simulink model "on_off_2022a"  (R2022a)
settings: Solver=ode4  StartTime=0.0  StopTime=1500  FixedStep=0.1  RelTol=1e-3  EnableMultiTasking=on
libraries: arduinolib x4
settings Model: ExtModeTrigDuration=2  Creator=user  LastModifiedBy=manur
settings SolverCC: AlgebraicLoopSolver=TrustRegion
settings DataIOCC: ReturnWorkspaceOutputs=off
settings OptimizationCC: EnhancedBackFolding=on  PassReuseOutputArgsAs=Individual arguments  MaxStackSize=64  OptimizeBlockOrder=speed  DifferentSizesBufferReuse=on  OptimizationCustomize=off  EfficientTunableParamExpr=on
settings DebuggingCC: ParameterTunabilityLossMsg=error  UnconnectedInputMsg=warning  UnconnectedOutputMsg=warning  UnconnectedLineMsg=warning  SFMachineParentedDataDiag=warning  ArithmeticOperatorsInVariantConditions=warning
settings HardwareCC: ProdBitPerInt=16  ProdBitPerPointer=16  ProdBitPerSizeT=16  ProdBitPerPtrDiffT=16  ProdLargestAtomicFloat=None  ProdWordSize=8  ProdHWDeviceType=Atmel->AVR
settings SFSimCC: SimUseLocalCustomCode=off  MATLABDynamicMemAlloc=off  CustomCodeUndefinedFunction=UseInterfaceOnly
settings SFSimCC: SimCustomInitializer=|
  | analogWrite(9, 0);
  | analogWrite(10, 0);
  | delay(1);
settings SFSimCC: SimCustomTerminator=|
  | analogWrite(9, 0);
  | analogWrite(10, 0);
  | delay(1);
settings RTWCC: SystemTargetFile=ert.tlc  HardwareBoard=Arduino Uno  TemplateMakefile=ert_default_tmf  GenerateReport=on  RTWUseLocalCustomCode=off  RTWUseSimCustomCode=on  Toolchain=Arduino AVR  BuildConfiguration=Faster Runs  IncludeHyperlinkInReport=on  LaunchReport=on  GenerateTraceInfo=on  GenerateTraceReport=on  GenerateTraceReportSl=on  GenerateTraceReportSf=on  GenerateTraceReportEml=on  DLArmComputeVersion=19.05
settings RTWCC: CustomInitializer=|
  | analogWrite(9, 0);
  | analogWrite(10, 0);
  | delay(1);
settings RTWCC: CustomTerminator=|
  | analogWrite(9, 0);
  | analogWrite(10, 0);
  | delay(1);
settings CodeAppCC: ForceParamTrailComments=on  IgnoreCustomStorageClasses=off  OperatorAnnotations=on  SimulinkDataObjDesc=on  SFDataObjDesc=on  InsertBlockDesc=on
settings ERTTargetCC: SupportContinuousTime=on  SupportVariableSizeSignals=on  ExtMode=on  ExtModeMexArgs='127.0.0.1' 0 17725

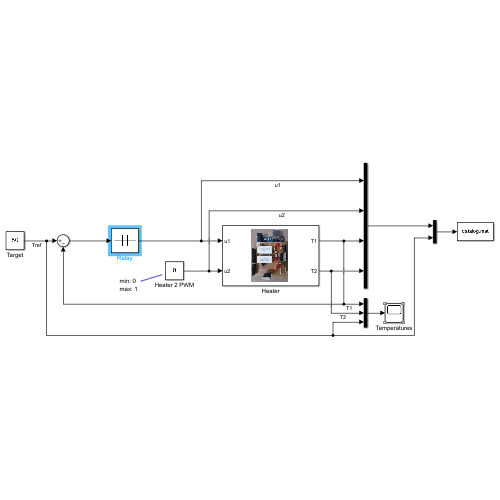
[thumbnail: Simulink's stored preview of the top-level diagram]
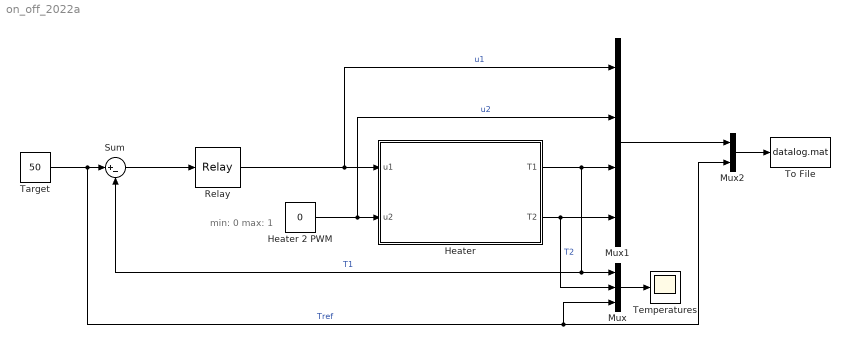
== system on_off_2022a ==
  note: min: 0
      | max: 1
  Heater : Subsystem
      mask Display: image('$imagefile'); % Use "Edit Image" on toolstrip to change.
  Heater 2 PWM : Constant  Value=0
  Mux : Mux  Inputs=3
  Mux1 : Mux
  Mux2 : Mux  Inputs=2
  Relay : Relay  OnSwitchValue=2  OffSwitchValue=-2  OnOutputValue=0.7
  Sum : Sum  Inputs=|+-
  Target : Constant  Value=50
  Temperatures : Scope
  To File : ToFile  Filename=datalog.mat  MatrixName=datalog
  wires:
  Mux1/1 -> Mux2/1
  Heater/2(T2) -> Mux/2, Mux1/4  "T2"
  Heater/1(T1) -> Mux/1, Sum/2, Mux1/3  "T1"
  Relay/1 -> Mux1/1, Heater/1(u1)  "u1"
  Mux/1 -> Temperatures/1
  Heater 2 PWM/1 -> Mux1/2, Heater/2(u2)  "u2"
  Sum/1 -> Relay/1
  Target/1 -> Mux2/2, Mux/3, Sum/1  "Tref"
  Mux2/1 -> To File/1

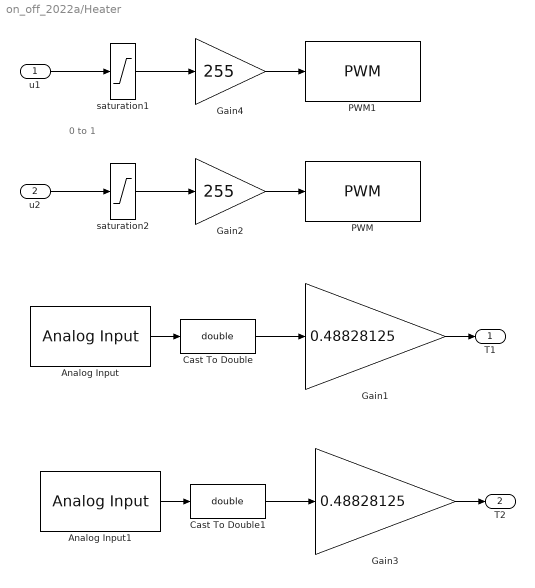
== system on_off_2022a/Heater ==
  note: 0 to 1
  u1 : Inport
  u2 : Inport  Port=2
  Analog Input : arduinolib/Analog Input  pinNumber=0  ReadResultsOnly=off  ConversionTriggerSource=Software  ExternalTriggerType=uint32(0)  OutputDataType=uint16  EnableConversionCompleteNotify=off  EnableOuputStatus=off  SampleTime=-1  blockPlatform=arduino
  Analog Input1 : arduinolib/Analog Input  pinNumber=1  ReadResultsOnly=off  ConversionTriggerSource=Software  ExternalTriggerType=uint32(0)  OutputDataType=uint16  EnableConversionCompleteNotify=off  EnableOuputStatus=off  SampleTime=-1  blockPlatform=arduino
  Cast To Double : DataTypeConversion  OutDataTypeStr=double  SaturateOnIntegerOverflow=off  RndMeth=Floor
  Cast To Double1 : DataTypeConversion  OutDataTypeStr=double  SaturateOnIntegerOverflow=off  RndMeth=Floor
  Gain1 : Gain  Gain=0.48828125
  Gain2 : Gain  Gain=255
  Gain3 : Gain  Gain=0.48828125
  Gain4 : Gain  Gain=255
  PWM : arduinolib/PWM  pinNumber=10  frequencyType=Default  desiredFrequency=980  achievableFrequency=980.0319
  PWM1 : arduinolib/PWM  pinNumber=9  frequencyType=Default  desiredFrequency=980  achievableFrequency=980.0319
  saturation1 : Saturate  UpperLimit=1  LowerLimit=0
  saturation2 : Saturate  UpperLimit=1  LowerLimit=0
  T1 : Outport  VectorParamsAs1DForOutWhenUnconnected=off
  T2 : Outport  Port=2  VectorParamsAs1DForOutWhenUnconnected=off
  wires:
  Gain1/1 -> T1/1
  Gain2/1 -> PWM/1
  Analog Input/1 -> Cast To Double/1
  Cast To Double/1 -> Gain1/1
  Cast To Double1/1 -> Gain3/1
  Gain3/1 -> T2/1
  Analog Input1/1 -> Cast To Double1/1
  Gain4/1 -> PWM1/1
  u1/1 -> saturation1/1
  u2/1 -> saturation2/1
  saturation1/1 -> Gain4/1
  saturation2/1 -> Gain2/1
